simulink model "EsamblajeCohete2_0"  (R2023a)
settings: Solver=VariableStepAuto  StartTime=0.0  StopTime=15  RelTol=1e-3
model workspace: external: MATLAB File C:\Users\SEBASTIANDIAZPABON\OneDrive - Universidad Santo Tomás Bucaramanga\USTA\Semillero Cohete\Cohete Matlab 2.0\EsamblajeCohete2_0_DataFile.m (data not in the file)
undefined symbols (not defined in the file): smiData, X, Y, Z
libraries: sm_lib x355, nesl_utility x10, fuzblock x6, simulink x2
(part 1 of 7)
settings Model: SimulationMode=accelerator  Creator=SEBASTIANDIAZPABON  LastModifiedBy=kushkiclave1234
settings ModelReferenceCC: EnableRefExpFcnMdlSchedulingChecks=on

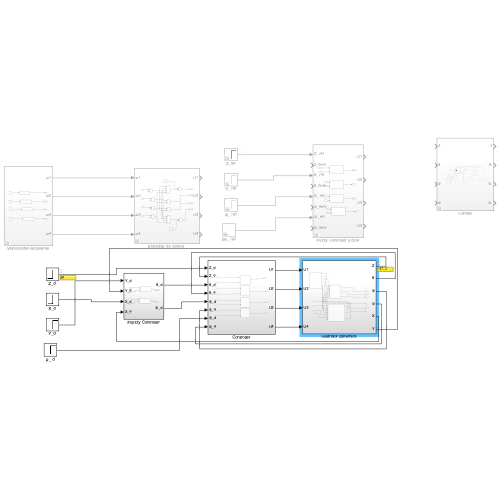
[thumbnail: Simulink's stored preview of the top-level diagram]
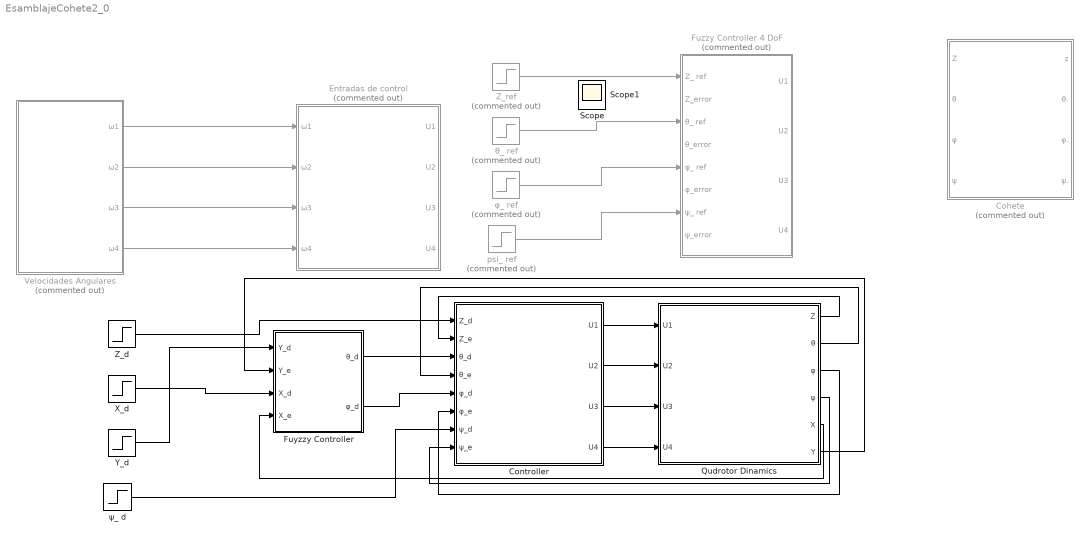
== system EsamblajeCohete2_0 ==
  Cohete : Subsystem  Commented=on
  Controller : Subsystem
  "Entradas de control " : Subsystem  Commented=on
  Fuyzzy Controller : Subsystem
  Fuzzy Controller 4 DoF : Subsystem  Commented=on
  Qudrotor Dinamics : Subsystem
  Velocidades Angulares : Subsystem  Commented=on
  X_d : Step  After=20  SampleTime=0
  Y_d : Step  After=20  SampleTime=0
  Z_d : Step  Time=0.01  After=30  SampleTime=0
  Z_ref : Step  Commented=on  Time=0  After=0  SampleTime=0
  psi_ ref : Step  Commented=on  Time=0  After=0.05  SampleTime=0
  θ_ ref : Step  Commented=on  Time=0  After=0.1  SampleTime=0
  φ_ ref : Step  Commented=on  Time=0  After=0.5  SampleTime=0
  ψ_ d : Step  After=20  SampleTime=0
  Scope : Scope
  Scope1 : Scope
  wires:
  Velocidades Angulares/1(ω1) -> "Entradas de control "/1(ω1)
  Velocidades Angulares/2(ω2) -> "Entradas de control "/2(ω2)
  Velocidades Angulares/3(ω3) -> "Entradas de control "/3(ω3)
  Velocidades Angulares/4(ω4) -> "Entradas de control "/4(ω4)
  Z_ref/1 -> Fuzzy Controller 4 DoF/1(Z_ ref)
  θ_ ref/1 -> Fuzzy Controller 4 DoF/3(θ_ ref)
  φ_ ref/1 -> Fuzzy Controller 4 DoF/5(φ_ ref)
  psi_ ref/1 -> Fuzzy Controller 4 DoF/7(ψ_ ref)
  Controller/1(U1) -> Qudrotor Dinamics/1(U1)
  Controller/2(U2) -> Qudrotor Dinamics/2(U2)
  Controller/3(U3) -> Qudrotor Dinamics/3(U3)
  Controller/4(U4) -> Qudrotor Dinamics/4(U4)
  Qudrotor Dinamics/1(Z) -> Controller/2(Z_e)
  Qudrotor Dinamics/2(θ) -> Controller/4(θ_e)
  Qudrotor Dinamics/3(φ) -> Controller/6(φ_e)
  Qudrotor Dinamics/4(ψ) -> Controller/8(ψ_e)
  Fuyzzy Controller/1(θ_d) -> Controller/3(θ_d)
  Qudrotor Dinamics/6(Y) -> Fuyzzy Controller/2(Y_e)
  Qudrotor Dinamics/5(X) -> Fuyzzy Controller/4(X_e)
  Fuyzzy Controller/2(φ_d) -> Controller/5(φ_d)
  Z_d/1 -> Controller/1(Z_d)
  X_d/1 -> Fuyzzy Controller/3(X_d)
  Y_d/1 -> Fuyzzy Controller/1(Y_d)
  ψ_ d/1 -> Controller/7(ψ_d)

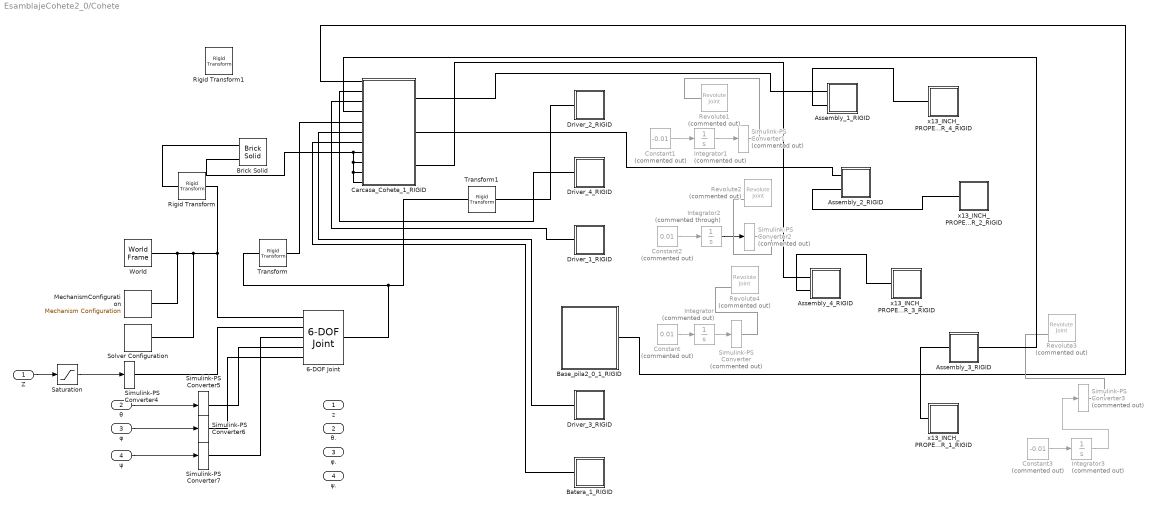
== system EsamblajeCohete2_0/Cohete ==
  Z : Inport
  θ : Inport  Port=2
  φ : Inport  Port=3
  ψ : Inport  Port=4
  6-DOF Joint : sm_lib/Joints/6-DOF Joint  JointMode=Normal  SenseConstraintForce=off  SenseConstraintForceX=off  SenseConstraintForceY=off  SenseConstraintForceZ=off  SenseConstraintTorque=off  SenseConstraintTorqueX=off  SenseConstraintTorqueY=off  SenseConstraintTorqueZ=off  SenseTotalForce=off  SenseTotalForceX=off  SenseTotalForceY=off  SenseTotalForceZ=off  SenseTotalTorque=off  SenseTotalTorqueX=off  SenseTotalTorqueY=off  SenseTotalTorqueZ=off  CompositeWrenchDir=FollowerOnBase  CompositeWrenchFrame=BaseFrame  PxEquilibriumPosition=0  PxEquilibriumPositionUnits=m  PxSpringStiffness=0  PxSpringStiffnessUnits=N/m  PxDampingCoefficient=0  PxDampingCoefficientUnits=N/(m/s)  PxTorqueActuationMode=NoTorque  PxMotionActuationMode=ComputedMotion  PxSensePosition=off  PxSenseVelocity=off  PxSenseAcceleration=off  PxSenseTorqueForce=off  PxSenseLowerLimitTorqueForce=off  PxSenseUpperLimitTorqueForce=off  PxLowerLimitSpecify=off  PxLowerLimitBound=-1  PxLowerLimitBoundUnits=m  PxLowerLimitStiffness=1e6  PxLowerLimitStiffnessUnits=N/m  PxLowerLimitDamping=1e3  PxLowerLimitDampingUnits=N/(m/s)  PxLowerLimitTransitionRegionWidth=1e-4  PxLowerLimitTransitionRegionWidthUnits=m  PxUpperLimitSpecify=off  PxUpperLimitBound=1  PxUpperLimitBoundUnits=m  PxUpperLimitStiffness=1e6  PxUpperLimitStiffnessUnits=N/m  PxUpperLimitDamping=1e3  PxUpperLimitDampingUnits=N/(m/s)  PxUpperLimitTransitionRegionWidth=1e-4  PxUpperLimitTransitionRegionWidthUnits=m  PxPositionTargetSpecify=off  PxPositionTargetPriority=High  PxPositionTargetValue=0  PxPositionTargetValueUnits=m  PxVelocityTargetSpecify=off  PxVelocityTargetPriority=High  PxVelocityTargetValue=0  PxVelocityTargetValueUnits=m/s  PyEquilibriumPosition=0  PyEquilibriumPositionUnits=m  PySpringStiffness=0  PySpringStiffnessUnits=N/m  PyDampingCoefficient=0  PyDampingCoefficientUnits=N/(m/s)  PyTorqueActuationMode=ComputedTorque  PyMotionActuationMode=InputMotion  PySensePosition=off  PySenseVelocity=off  PySenseAcceleration=off  PySenseTorqueForce=off  PySenseLowerLimitTorqueForce=off  PySenseUpperLimitTorqueForce=off  PyLowerLimitSpecify=on  PyLowerLimitBound=0  PyLowerLimitBoundUnits=m  PyLowerLimitStiffness=1e6  PyLowerLimitStiffnessUnits=N/m  PyLowerLimitDamping=1e3  PyLowerLimitDampingUnits=N/(m/s)  PyLowerLimitTransitionRegionWidth=1e-4  PyLowerLimitTransitionRegionWidthUnits=m  PyUpperLimitSpecify=off  PyUpperLimitBound=1  PyUpperLimitBoundUnits=m  PyUpperLimitStiffness=1e6  PyUpperLimitStiffnessUnits=N/m  PyUpperLimitDamping=1e3  PyUpperLimitDampingUnits=N/(m/s)  PyUpperLimitTransitionRegionWidth=1e-4  PyUpperLimitTransitionRegionWidthUnits=m  PyPositionTargetSpecify=off  PyPositionTargetPriority=High  PyPositionTargetValue=0  PyPositionTargetValueUnits=m  PyVelocityTargetSpecify=off  PyVelocityTargetPriority=High  PyVelocityTargetValue=0  PyVelocityTargetValueUnits=m/s  PzEquilibriumPosition=0  PzEquilibriumPositionUnits=m  PzSpringStiffness=0  PzSpringStiffnessUnits=N/m  PzDampingCoefficient=0  PzDampingCoefficientUnits=N/(m/s)  PzTorqueActuationMode=NoTorque  PzMotionActuationMode=ComputedMotion  PzSensePosition=off  PzSenseVelocity=off  PzSenseAcceleration=off  PzSenseTorqueForce=off  PzSenseLowerLimitTorqueForce=off  PzSenseUpperLimitTorqueForce=off  PzLowerLimitSpecify=off  PzLowerLimitBound=-1  PzLowerLimitBoundUnits=m  PzLowerLimitStiffness=1e6  PzLowerLimitStiffnessUnits=N/m  PzLowerLimitDamping=1e3  PzLowerLimitDampingUnits=N/(m/s)  PzLowerLimitTransitionRegionWidth=1e-4  PzLowerLimitTransitionRegionWidthUnits=m  PzUpperLimitSpecify=off  PzUpperLimitBound=1  PzUpperLimitBoundUnits=m  PzUpperLimitStiffness=1e6  PzUpperLimitStiffnessUnits=N/m  PzUpperLimitDamping=1e3  PzUpperLimitDampingUnits=N/(m/s)  PzUpperLimitTransitionRegionWidth=1e-4  PzUpperLimitTransitionRegionWidthUnits=m  PzPositionTargetSpecify=off  PzPositionTargetPriority=High  PzPositionTargetValue=0  PzPositionTargetValueUnits=m  PzVelocityTargetSpecify=off  PzVelocityTargetPriority=High  PzVelocityTargetValue=0  PzVelocityTargetValueUnits=m/s  SphEqPosRotationMethod=None  SphEqPosRotationAngleUnits=deg  SphEqPosRotationStandardAxis=+Z  SphEqPosRotationAngle=0.0  SphEqPosRotationArbitraryAxis=[0 0 1]  SphEqPosFollAlignAxisA=+X  SphEqPosBaseAlignAxisA=+Y  SphEqPosFollAlignAxisB=+Y  SphEqPosBaseAlignAxisB=+Z  SphEqPosRotationSequenceAxes=FollowerAxes  SphEqPosRotationSequence=XYX  SphEqPosRotationSequenceAngles=[0 0 0]  SphEqPosRotationSequenceAnglesUnits=deg  SphEqPosRotationMatrix=[1 0 0; 0 1 0; 0 0 1]  SphEqPosQuaternion=[1 0 0 0]  SphSpringStiffness=0  SphSpringStiffnessUnits=N*m/deg  SphDampingCoefficient=0  SphDampingCoefficientUnits=N*m/(deg/s)  SphActuateTorqueX=on  SphActuateTorqueY=on  SphActuateTorqueZ=on  SphActuateTorque=off  SphTorqueActuationMode=InputTorque  SphMotionActuationMode=ComputedMotion  SphActuationFrame=BaseFrame  SphSensePosition=off  SphSenseVelocityX=off  SphSenseVelocityY=off  SphSenseVelocityZ=off  SphSenseVelocity=off  SphSenseAccelerationX=off  SphSenseAccelerationY=off  SphSenseAccelerationZ=off  SphSenseAcceleration=off  SphSenseTorqueX=off  SphSenseTorqueY=off  SphSenseTorqueZ=off  SphSenseTorqueForce=off  SphSenseLowerLimitTorqueMag=off  SphSenseUpperLimitTorqueMag=off  SphSensingFrame=BaseFrame  SphLowerLimitSpecify=off  SphLowerLimitBound=15  SphLowerLimitBoundUnits=deg  SphLowerLimitStiffness=1e4  SphLowerLimitStiffnessUnits=N*m/deg  SphLowerLimitDamping=10  SphLowerLimitDampingUnits=N*m/(deg/s)  SphLowerLimitTransitionRegionWidth=0.1  SphLowerLimitTransitionRegionWidthUnits=deg  SphUpperLimitSpecify=off  SphUpperLimitBound=45  SphUpperLimitBoundUnits=deg  SphUpperLimitStiffness=1e4  SphUpperLimitStiffnessUnits=N*m/deg  SphUpperLimitDamping=10  SphUpperLimitDampingUnits=N*m/(deg/s)  SphUpperLimitTransitionRegionWidth=0.1  SphUpperLimitTransitionRegionWidthUnits=deg  SphPositionTargetRotationMethod=None  SphPositionTargetRotationAngleUnits=deg  SphPositionTargetRotationStandardAxis=+Z  SphPositionTargetRotationAngle=0.0  SphPositionTargetRotationArbitraryAxis=[0 0 1]  SphPositionTargetFollAlignAxisA=+X  SphPositionTargetBaseAlignAxisA=+Y  SphPositionTargetFollAlignAxisB=+Y  SphPositionTargetBaseAlignAxisB=+Z  SphPositionTargetRotationSequenceAxes=FollowerAxes  SphPositionTargetRotationSequence=XYX  SphPositionTargetRotationSequenceAngles=[0 0 0]  SphPositionTargetRotationSequenceAnglesUnits=deg  SphPositionTargetRotationMatrix=[1 0 0; 0 1 0; 0 0 1]  SphPositionTargetQuaternion=[1 0 0 0]  SphPositionTargetSpecify=off  SphPositionTargetPriority=High  SphVelocityTargetValue=[0 0 0]  SphVelocityTargetValueUnits=deg/s  SphVelocityTargetSpecify=off  SphVelocityTargetPriority=High  SphVelocityTargetInFollowerFrame=on
  Assembly_1_RIGID : Subsystem
  Assembly_2_RIGID : Subsystem
  Assembly_3_RIGID : Subsystem
  Assembly_4_RIGID : Subsystem
  Base_pila2_0_1_RIGID : Subsystem
  Batera_1_RIGID : Subsystem
  Brick Solid : sm_lib/Body Elements/Brick Solid  GraphicAmbientColor=[0.15 0.15 0.15 1.0]  BasedOnType=Density  BrickDimensions=[2 2 0.1 ]  BrickDimensionsUnits=m  CenterOfMass=[0 0 0]  CenterOfMassUnits=m  GraphicDiffuseColor=[0.4 0.6 0.0]  Density=1000  DensityUnits=kg/m^3  DoExposeReferenceFrame=on  GraphicEmissiveColor=[0.0 0.0 0.0 1.0]  ExportEntireGeometry=on  SerializedFrames=<Frames><Frame><Id>Frame1</Id><Value><Name>F1</Name><Origin><Source>ReferenceFrame</Source><FeatureName></FeatureName></Origin><PrimaryAxis><DefinedDirection>+Y</DefinedDirection><Source>ReferenceFrame</Source><SourceDirection>-Z</SourceDirection><FeatureName></FeatureName></PrimaryAxis><SecondaryAxis><DefinedDirection>+X</DefinedDirection><Source>ReferenceFrame</Source><SourceDirection>+X</SourceDirection><FeatureName></FeatureName></SecondaryAxis></Value></Frame></Frames>  MarkerShape=Sphere  MarkerSize=10  GraphicType=FromGeometry  InertiaType=CalculateFromGeometry  Mass=1  MassUnits=kg  MomentsOfInertia=[1 1 1]  MomentsOfInertiaUnits=kg*m^2  GraphicOpacity=1.0  ProductsOfInertia=[0 0 0]  ProductsOfInertiaUnits=kg*m^2  GraphicShininess=75  GraphicSpecularColor=[0.5 0.5 0.5 1.0]  GraphicVisPropType=SimpleVisualProperties
  Carcasa_Cohete_1_RIGID : Subsystem
  Constant : Constant  Commented=on  Value=0.01
  Constant1 : Constant  Commented=on  Value=-0.01
  Constant2 : Constant  Commented=on  Value=0.01
  Constant3 : Constant  Commented=on  Value=-0.01
  Driver_1_RIGID : Subsystem
  Driver_2_RIGID : Subsystem
  Driver_3_RIGID : Subsystem
  Driver_4_RIGID : Subsystem
  Integrator : Integrator  Commented=on
  Integrator1 : Integrator  Commented=on
  Integrator2 : Integrator  Commented=through
  Integrator3 : Integrator  Commented=on
  MechanismConfiguration : sm_lib/Utilities/Mechanism Configuration  UniformGravity=Constant  GravityVector=[0 0 0]  GravityVectorUnits=m/s^2  LinearizationDelta=0.001  JointModeTransitionNonlinearIterations=2
  Revolute1 : sm_lib/Joints/Revolute Joint  Commented=on  JointMode=Normal  SenseConstraintForce=off  SenseConstraintForceX=off  SenseConstraintForceY=off  SenseConstraintForceZ=off  SenseConstraintTorque=off  SenseConstraintTorqueX=off  SenseConstraintTorqueY=off  SenseConstraintTorqueZ=off  SenseTotalForce=off  SenseTotalForceX=off  SenseTotalForceY=off  SenseTotalForceZ=off  SenseTotalTorque=off  SenseTotalTorqueX=off  SenseTotalTorqueY=off  SenseTotalTorqueZ=off  CompositeWrenchDir=FollowerOnBase  CompositeWrenchFrame=BaseFrame  EquilibriumPosition=0  EquilibriumPositionUnits=deg  SpringStiffness=0  SpringStiffnessUnits=N*m/deg  DampingCoefficient=0  DampingCoefficientUnits=N*m/(deg/s)  TorqueActuationMode=InputTorque  MotionActuationMode=InputMotion  SensePosition=off  SenseVelocity=off  SenseAcceleration=off  SenseTorqueForce=off  SenseLowerLimitTorqueForce=off  SenseUpperLimitTorqueForce=off  LowerLimitSpecify=off  LowerLimitBound=-90  LowerLimitBoundUnits=deg  LowerLimitStiffness=1e4  LowerLimitStiffnessUnits=N*m/deg  LowerLimitDamping=10  LowerLimitDampingUnits=N*m/(deg/s)  LowerLimitTransitionRegionWidth=0.1  LowerLimitTransitionRegionWidthUnits=deg  UpperLimitSpecify=off  UpperLimitBound=90  UpperLimitBoundUnits=deg  UpperLimitStiffness=1e4  UpperLimitStiffnessUnits=N*m/deg  UpperLimitDamping=10  UpperLimitDampingUnits=N*m/(deg/s)  UpperLimitTransitionRegionWidth=0.1  UpperLimitTransitionRegionWidthUnits=deg  PositionTargetSpecify=on  PositionTargetPriority=Low  PositionTargetValue=smiData.RevoluteJoint(2).Rz.Pos  PositionTargetValueUnits=deg  VelocityTargetSpecify=off  VelocityTargetPriority=High  VelocityTargetValue=0  VelocityTargetValueUnits=deg/s
  Revolute2 : sm_lib/Joints/Revolute Joint  Commented=on  JointMode=Normal  SenseConstraintForce=off  SenseConstraintForceX=off  SenseConstraintForceY=off  SenseConstraintForceZ=off  SenseConstraintTorque=off  SenseConstraintTorqueX=off  SenseConstraintTorqueY=off  SenseConstraintTorqueZ=off  SenseTotalForce=off  SenseTotalForceX=off  SenseTotalForceY=off  SenseTotalForceZ=off  SenseTotalTorque=off  SenseTotalTorqueX=off  SenseTotalTorqueY=off  SenseTotalTorqueZ=off  CompositeWrenchDir=FollowerOnBase  CompositeWrenchFrame=BaseFrame  EquilibriumPosition=0  EquilibriumPositionUnits=deg  SpringStiffness=0  SpringStiffnessUnits=N*m/deg  DampingCoefficient=0  DampingCoefficientUnits=N*m/(deg/s)  TorqueActuationMode=InputTorque  MotionActuationMode=ComputedMotion  SensePosition=off  SenseVelocity=off  SenseAcceleration=off  SenseTorqueForce=off  SenseLowerLimitTorqueForce=off  SenseUpperLimitTorqueForce=off  LowerLimitSpecify=off  LowerLimitBound=-90  LowerLimitBoundUnits=deg  LowerLimitStiffness=1e4  LowerLimitStiffnessUnits=N*m/deg  LowerLimitDamping=10  LowerLimitDampingUnits=N*m/(deg/s)  LowerLimitTransitionRegionWidth=0.1  LowerLimitTransitionRegionWidthUnits=deg  UpperLimitSpecify=off  UpperLimitBound=90  UpperLimitBoundUnits=deg  UpperLimitStiffness=1e4  UpperLimitStiffnessUnits=N*m/deg  UpperLimitDamping=10  UpperLimitDampingUnits=N*m/(deg/s)  UpperLimitTransitionRegionWidth=0.1  UpperLimitTransitionRegionWidthUnits=deg  PositionTargetSpecify=on  PositionTargetPriority=Low  PositionTargetValue=smiData.RevoluteJoint(3).Rz.Pos  PositionTargetValueUnits=deg  VelocityTargetSpecify=off  VelocityTargetPriority=High  VelocityTargetValue=0  VelocityTargetValueUnits=deg/s
  Revolute3 : sm_lib/Joints/Revolute Joint  Commented=on  JointMode=Normal  SenseConstraintForce=off  SenseConstraintForceX=off  SenseConstraintForceY=off  SenseConstraintForceZ=off  SenseConstraintTorque=off  SenseConstraintTorqueX=off  SenseConstraintTorqueY=off  SenseConstraintTorqueZ=off  SenseTotalForce=off  SenseTotalForceX=off  SenseTotalForceY=off  SenseTotalForceZ=off  SenseTotalTorque=off  SenseTotalTorqueX=off  SenseTotalTorqueY=off  SenseTotalTorqueZ=off  CompositeWrenchDir=FollowerOnBase  CompositeWrenchFrame=BaseFrame  EquilibriumPosition=0  EquilibriumPositionUnits=deg  SpringStiffness=0  SpringStiffnessUnits=N*m/deg  DampingCoefficient=0  DampingCoefficientUnits=N*m/(deg/s)  TorqueActuationMode=InputTorque  MotionActuationMode=ComputedMotion  SensePosition=off  SenseVelocity=off  SenseAcceleration=off  SenseTorqueForce=off  SenseLowerLimitTorqueForce=off  SenseUpperLimitTorqueForce=off  LowerLimitSpecify=off  LowerLimitBound=-90  LowerLimitBoundUnits=deg  LowerLimitStiffness=1e4  LowerLimitStiffnessUnits=N*m/deg  LowerLimitDamping=10  LowerLimitDampingUnits=N*m/(deg/s)  LowerLimitTransitionRegionWidth=0.1  LowerLimitTransitionRegionWidthUnits=deg  UpperLimitSpecify=off  UpperLimitBound=90  UpperLimitBoundUnits=deg  UpperLimitStiffness=1e4  UpperLimitStiffnessUnits=N*m/deg  UpperLimitDamping=10  UpperLimitDampingUnits=N*m/(deg/s)  UpperLimitTransitionRegionWidth=0.1  UpperLimitTransitionRegionWidthUnits=deg  PositionTargetSpecify=on  PositionTargetPriority=Low  PositionTargetValue=smiData.RevoluteJoint(4).Rz.Pos  PositionTargetValueUnits=deg  VelocityTargetSpecify=off  VelocityTargetPriority=High  VelocityTargetValue=0  VelocityTargetValueUnits=deg/s
  Revolute4 : sm_lib/Joints/Revolute Joint  Commented=on  JointMode=Normal  SenseConstraintForce=off  SenseConstraintForceX=off  SenseConstraintForceY=off  SenseConstraintForceZ=off  SenseConstraintTorque=off  SenseConstraintTorqueX=off  SenseConstraintTorqueY=off  SenseConstraintTorqueZ=off  SenseTotalForce=off  SenseTotalForceX=off  SenseTotalForceY=off  SenseTotalForceZ=off  SenseTotalTorque=off  SenseTotalTorqueX=off  SenseTotalTorqueY=off  SenseTotalTorqueZ=off  CompositeWrenchDir=FollowerOnBase  CompositeWrenchFrame=BaseFrame  EquilibriumPosition=0  EquilibriumPositionUnits=deg  SpringStiffness=0  SpringStiffnessUnits=N*m/deg  DampingCoefficient=0  DampingCoefficientUnits=N*m/(deg/s)  TorqueActuationMode=InputTorque  MotionActuationMode=ComputedMotion  SensePosition=off  SenseVelocity=off  SenseAcceleration=off  SenseTorqueForce=off  SenseLowerLimitTorqueForce=off  SenseUpperLimitTorqueForce=off  LowerLimitSpecify=off  LowerLimitBound=-90  LowerLimitBoundUnits=deg  LowerLimitStiffness=1e4  LowerLimitStiffnessUnits=N*m/deg  LowerLimitDamping=10  LowerLimitDampingUnits=N*m/(deg/s)  LowerLimitTransitionRegionWidth=0.1  LowerLimitTransitionRegionWidthUnits=deg  UpperLimitSpecify=off  UpperLimitBound=90  UpperLimitBoundUnits=deg  UpperLimitStiffness=1e4  UpperLimitStiffnessUnits=N*m/deg  UpperLimitDamping=10  UpperLimitDampingUnits=N*m/(deg/s)  UpperLimitTransitionRegionWidth=0.1  UpperLimitTransitionRegionWidthUnits=deg  PositionTargetSpecify=on  PositionTargetPriority=Low  PositionTargetValue=smiData.RevoluteJoint(5).Rz.Pos  PositionTargetValueUnits=deg  VelocityTargetSpecify=off  VelocityTargetPriority=High  VelocityTargetValue=0  VelocityTargetValueUnits=deg/s
  Rigid Transform : sm_lib/Frames and Transforms/Rigid Transform  TranslationMethod=Cartesian  TranslationStandardOffset=0  TranslationStandardOffsetUnits=m  TranslationStandardAxis=+Z  TranslationCartesianOffset=[0 0.28 0]  TranslationCartesianOffsetUnits=m  TranslationROffset=0  TranslationROffsetUnits=m  TranslationZOffset=0  TranslationZOffsetUnits=m  TranslationThetaOffset=0  TranslationThetaOffsetUnits=deg  RotationMethod=None  RotationAngleUnits=deg  RotationStandardAxis=+Z  RotationAngle=0.0  RotationArbitraryAxis=[0 0 1]  FollAlignAxisA=+X  BaseAlignAxisA=+Y  FollAlignAxisB=+Y  BaseAlignAxisB=+Z  RotationSequenceAxes=FollowerAxes  RotationSequence=XYX  RotationSequenceAngles=[0 0 0]  RotationSequenceAnglesUnits=deg  RotationMatrix=[1 0 0; 0 1 0; 0 0 1]  Quaternion=[1 0 0 0]
  Rigid Transform1 : sm_lib/Frames and Transforms/Rigid Transform  TranslationMethod=None  TranslationStandardOffset=0  TranslationStandardOffsetUnits=m  TranslationStandardAxis=+Z  TranslationCartesianOffset=[0 0 0]  TranslationCartesianOffsetUnits=m  TranslationROffset=0  TranslationROffsetUnits=m  TranslationZOffset=0  TranslationZOffsetUnits=m  TranslationThetaOffset=0  TranslationThetaOffsetUnits=deg  RotationMethod=None  RotationAngleUnits=deg  RotationStandardAxis=+Z  RotationAngle=0.0  RotationArbitraryAxis=[0 0 1]  FollAlignAxisA=+X  BaseAlignAxisA=+Y  FollAlignAxisB=+Y  BaseAlignAxisB=+Z  RotationSequenceAxes=FollowerAxes  RotationSequence=XYX  RotationSequenceAngles=[0 0 0]  RotationSequenceAnglesUnits=deg  RotationMatrix=[1 0 0; 0 1 0; 0 0 1]  Quaternion=[1 0 0 0]
  Saturation : Saturate  UpperLimit=2  LowerLimit=-2
  Simulink-PS Converter{,1..3} (4 alike) : nesl_utility/Simulink-PS Converter  Commented=on  PhysicalDomain=network_engine_domain  SubClassName=ps_input  LeftPortType=input  RightPortType=output  PseudoPeriodic=off  Frequencies=[]  NoiseDistribution=none  NoiseParameters=[]  Unit=1  AffineConversion=off  FilteringAndDerivatives=filter  SimscapeFilterOrder=2  InputFilterTimeConstant=0.001  UdotUserProvided=0
  Simulink-PS Converter{4..7} (4 alike) : nesl_utility/Simulink-PS Converter  PhysicalDomain=network_engine_domain  SubClassName=ps_input  LeftPortType=input  RightPortType=output  PseudoPeriodic=off  Frequencies=[]  NoiseDistribution=none  NoiseParameters=[]  Unit=1  AffineConversion=off  FilteringAndDerivatives=filter  SimscapeFilterOrder=2  InputFilterTimeConstant=0.001  UdotUserProvided=0
  Solver Configuration : nesl_utility/Solver Configuration  PhysicalDomain=network_engine_domain  SubClassName=solver  LeftPortType=input  RightPortType=generic  Tones=[]  Harmonics=[]  SimulateNoise=off  Profile=off  UseLocalSampling=off  EnableSwitchedLinearOptims=on  FrequencyDomain=off  UseCCode=off  RelTol=0.001  AbsTol=0.001  MinStep=1e-09  ToWorkspace=off  RevertToSquareIcSolve=off  NumHomotopyIterations=100  PhasorMode=off  PhasorModeNumHarmonics=1  ConsistencySolver=NEWTON_FTOL  IndexReductionMethod=DerivativeReplacement  DoDC=off  ResidualTolerance=1e-09  ConsistencyTolSource=GLOBAL  ConsistencyAbsTol=0.001  ConsistencyRelTol=0.001  ConsistencyTolFactor=0.001  UseLocalSolver=off  LocalSolverChoice=NE_BACKWARD_EULER_ADVANCER  ResolveIndetEquations=on  FunctionEvalNumThread=1  LocalSolverSampleTime=0.001  DoFixedCost=off  MaxNonlinIter=3  MaxModeIter=2  ComputeImpulses=off  ImpulseIterations=2  LinearAlgebra=auto  LinearAlgebraNumThread=0  EquationFormulation=NE_TIME_EF  DelaysMemoryBudget=1024  AutomaticFiltering=on  FilteringTimeConstant=0.001  PartitionStorageMethod=AS_NEEDED  PartitionMemoryBudget=1024  PartitionMethod=ROBUST
  Transform : sm_lib/Frames and Transforms/Rigid Transform  TranslationMethod=Cartesian  TranslationStandardOffset=0  TranslationStandardOffsetUnits=mm  TranslationStandardAxis=+Z  TranslationCartesianOffset=smiData.RigidTransform(12).translation  TranslationCartesianOffsetUnits=mm  TranslationROffset=0  TranslationROffsetUnits=m  TranslationZOffset=0  TranslationZOffsetUnits=m  TranslationThetaOffset=0  TranslationThetaOffsetUnits=deg  RotationMethod=ArbitraryAxis  RotationAngleUnits=rad  RotationStandardAxis=+Z  RotationAngle=smiData.RigidTransform(12).angle  RotationArbitraryAxis=smiData.RigidTransform(12).axis  FollAlignAxisA=+X  BaseAlignAxisA=+Y  FollAlignAxisB=+Y  BaseAlignAxisB=+Z  RotationSequenceAxes=FollowerAxes  RotationSequence=XYX  RotationSequenceAngles=[0 0 0]  RotationSequenceAnglesUnits=deg  RotationMatrix=[1 0 0; 0 1 0; 0 0 1]  Quaternion=[1 0 0 0]
  Transform1 : sm_lib/Frames and Transforms/Rigid Transform  TranslationMethod=Cartesian  TranslationStandardOffset=0  TranslationStandardOffsetUnits=mm  TranslationStandardAxis=+Z  TranslationCartesianOffset=smiData.RigidTransform(123).translation  TranslationCartesianOffsetUnits=mm  TranslationROffset=0  TranslationROffsetUnits=m  TranslationZOffset=0  TranslationZOffsetUnits=m  TranslationThetaOffset=0  TranslationThetaOffsetUnits=deg  RotationMethod=ArbitraryAxis  RotationAngleUnits=rad  RotationStandardAxis=+Z  RotationAngle=smiData.RigidTransform(123).angle  RotationArbitraryAxis=smiData.RigidTransform(123).axis  FollAlignAxisA=+X  BaseAlignAxisA=+Y  FollAlignAxisB=+Y  BaseAlignAxisB=+Z  RotationSequenceAxes=FollowerAxes  RotationSequence=XYX  RotationSequenceAngles=[0 0 0]  RotationSequenceAnglesUnits=deg  RotationMatrix=[1 0 0; 0 1 0; 0 0 1]  Quaternion=[1 0 0 0]
  World : sm_lib/Frames and Transforms/World Frame
  x13_INCH_PROPELLER_1_RIGID : Subsystem
  x13_INCH_PROPELLER_2_RIGID : Subsystem
  x13_INCH_PROPELLER_3_RIGID : Subsystem
  x13_INCH_PROPELLER_4_RIGID : Subsystem
  z : Outport
  θ. : Outport  Port=2
  φ. : Outport  Port=3
  ψ. : Outport  Port=4
  wires:
  θ/1 -> Simulink-PS Converter5/1
  φ/1 -> Simulink-PS Converter6/1
  Z/1 -> Saturation/1
  Integrator3/1 -> Simulink-PS Converter3/1
  Integrator1/1 -> Simulink-PS Converter1/1
  Integrator2/1 -> Simulink-PS Converter2/1
  Constant3/1 -> Integrator3/1
  Constant/1 -> Integrator/1
  Constant1/1 -> Integrator1/1
  Constant2/1 -> Integrator2/1
  Integrator/1 -> Simulink-PS Converter/1
  ψ/1 -> Simulink-PS Converter7/1
  Saturation/1 -> Simulink-PS Converter4/1
  connections:
  Driver_2_RIGID/LConn1 -- Transform1/RConn1
  Assembly_3_RIGID/LConn1 -- x13_INCH_PROPELLER_1_RIGID/LConn1
  Revolute1/LConn2 -- Simulink-PS Converter1/RConn1
  Transform/RConn1 -- Carcasa_Cohete_1_RIGID/LConn5
  Base_pila2_0_1_RIGID/RConn1 -- Carcasa_Cohete_1_RIGID/LConn1
  Assembly_4_RIGID/LConn2 -- x13_INCH_PROPELLER_3_RIGID/LConn1
  Simulink-PS Converter2/RConn1 -- Revolute2/LConn2
  Revolute3/LConn2 -- Simulink-PS Converter3/RConn1
  Transform1/LConn1 -- Transform/LConn1 -- 6-DOF Joint/RConn1
  Simulink-PS Converter/RConn1 -- Revolute4/LConn2
  Batera_1_RIGID/LConn1 -- Carcasa_Cohete_1_RIGID/LConn7
  Assembly_1_RIGID/LConn2 -- x13_INCH_PROPELLER_4_RIGID/LConn1
  Driver_4_RIGID/LConn1 -- Carcasa_Cohete_1_RIGID/LConn2
  Driver_3_RIGID/LConn1 -- Carcasa_Cohete_1_RIGID/LConn6
  Driver_1_RIGID/LConn1 -- Carcasa_Cohete_1_RIGID/LConn3
  Assembly_2_RIGID/LConn2 -- x13_INCH_PROPELLER_2_RIGID/LConn1
  Brick Solid/LConn2 -- Carcasa_Cohete_1_RIGID/LConn11 -- Carcasa_Cohete_1_RIGID/LConn10 -- Carcasa_Cohete_1_RIGID/LConn9 -- Carcasa_Cohete_1_RIGID/LConn8
  Simulink-PS Converter4/RConn1 -- 6-DOF Joint/LConn2
  Carcasa_Cohete_1_RIGID/RConn2 -- Assembly_2_RIGID/LConn1
  Carcasa_Cohete_1_RIGID/RConn1 -- Assembly_1_RIGID/LConn1
  Carcasa_Cohete_1_RIGID/RConn3 -- Assembly_4_RIGID/LConn1
  Carcasa_Cohete_1_RIGID/LConn4 -- Assembly_3_RIGID/RConn1
  MechanismConfiguration/RConn1 -- World/RConn1 -- Rigid Transform/RConn1 -- 6-DOF Joint/LConn1 -- Solver Configuration/RConn1
  Rigid Transform/LConn1 -- Brick Solid/LConn1
  Simulink-PS Converter7/RConn1 -- 6-DOF Joint/LConn3
  Simulink-PS Converter5/RConn1 -- 6-DOF Joint/LConn4
  Simulink-PS Converter6/RConn1 -- 6-DOF Joint/LConn5

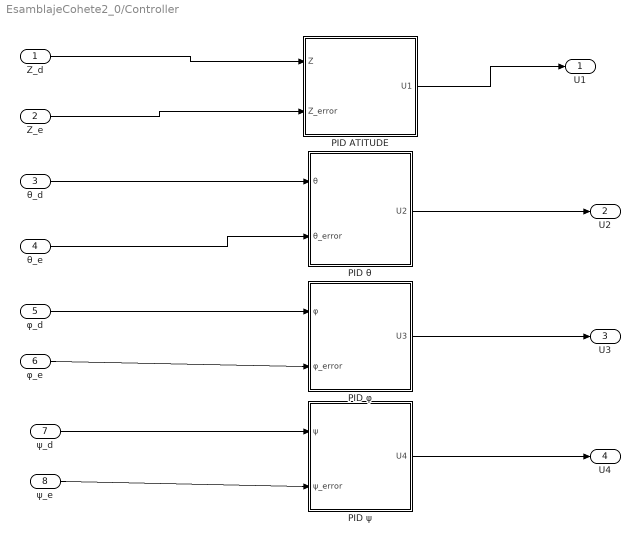
== system EsamblajeCohete2_0/Controller ==
  Z_d : Inport
  Z_e : Inport  Port=2
  θ_d : Inport  Port=3
  θ_e : Inport  Port=4
  φ_d : Inport  Port=5
  φ_e : Inport  Port=6
  ψ_d : Inport  Port=7
  ψ_e : Inport  Port=8
  PID ATITUDE : Subsystem
  "PID θ   " : Subsystem
  PID φ : Subsystem
  PID ψ : Subsystem
  U1 : Outport
  U2 : Outport  Port=2
  U3 : Outport  Port=3
  U4 : Outport  Port=4
  wires:
  PID ATITUDE/1(U1) -> U1/1
  "PID θ   "/1(U2) -> U2/1
  Z_d/1 -> PID ATITUDE/1(Z)
  Z_e/1 -> PID ATITUDE/2(Z_error)
  θ_d/1 -> "PID θ   "/1(θ)
  θ_e/1 -> "PID θ   "/2(θ_error)
  φ_d/1 -> PID φ/1(φ)
  φ_e/1 -> PID φ/2(φ_error)
  PID φ/1(U3) -> U3/1
  PID ψ/1(U4) -> U4/1
  ψ_d/1 -> PID ψ/1(ψ)
  ψ_e/1 -> PID ψ/2(ψ_error)

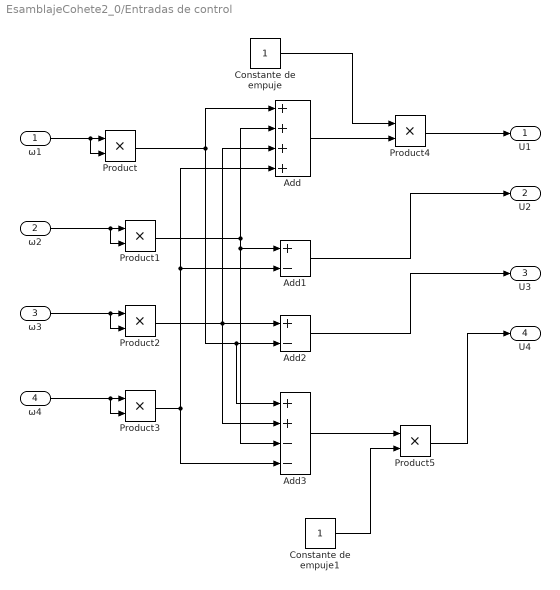
== system EsamblajeCohete2_0/Entradas de control  ==
  ω1 : Inport
  ω2 : Inport  Port=2
  ω3 : Inport  Port=3
  ω4 : Inport  Port=4
  Add : Sum  Inputs=++++
  Add1 : Sum  Inputs=+-
  Add2 : Sum  Inputs=+-
  Add3 : Sum  Inputs=++--
  Constante de empuje : Constant
  Constante de empuje1 : Constant
  Product{,1..5} (6 alike) : Product
  U1 : Outport
  U2 : Outport  Port=2
  U3 : Outport  Port=3
  U4 : Outport  Port=4
  wires:
  ω1/1 -> Product/2, Product/1
  ω2/1 -> Product1/2, Product1/1
  ω3/1 -> Product2/2, Product2/1
  ω4/1 -> Product3/2, Product3/1
  Product/1 -> Add3/1, Add2/2, Add/1
  Product1/1 -> Add1/1, Add3/3, Add/2
  Product2/1 -> Add2/1, Add/3, Add3/2
  Product3/1 -> Add3/4, Add1/2, Add/4
  Add/1 -> Product4/2
  Constante de empuje/1 -> Product4/1
  Product4/1 -> U1/1
  Add1/1 -> U2/1
  Add2/1 -> U3/1
  Add3/1 -> Product5/1
  Constante de empuje1/1 -> Product5/2
  Product5/1 -> U4/1

== system EsamblajeCohete2_0/Fuyzzy Controller ==
  Y_d : Inport
  Y_e : Inport  Port=2
  X_d : Inport  Port=3
  X_e : Inport  Port=4
  Fuzzy Lateral Controller : Subsystem
  Fuzzy Longitudinal Controller : Subsystem
  θ_d : Outport
  φ_d : Outport  Port=2
  wires:
  Y_d/1 -> Fuzzy Longitudinal Controller/1(Y_d)
  Fuzzy Longitudinal Controller/1(θ_d) -> θ_d/1
  Y_e/1 -> Fuzzy Longitudinal Controller/2(Y_e)
  X_d/1 -> Fuzzy Lateral Controller/1(X_d)
  Fuzzy Lateral Controller/1(θ_d) -> φ_d/1
  X_e/1 -> Fuzzy Lateral Controller/2(X_e)

== system EsamblajeCohete2_0/Fuzzy Controller 4 DoF ==
  Z_ ref : Inport
  Z_error : Inport  Port=2
  θ_ ref : Inport  Port=3
  θ_error : Inport  Port=4
  φ_ ref : Inport  Port=5
  φ_error : Inport  Port=6
  ψ_ ref : Inport  Port=7
  ψ_error : Inport  Port=8
  Fuzzy Controller Z : Subsystem
  Fuzzy Controller θ : Subsystem
  Fuzzy Controller φ : Subsystem
  Fuzzy Controller ψ : Subsystem
  U1 : Outport
  U2 : Outport  Port=2
  U3 : Outport  Port=3
  U4 : Outport  Port=4
  wires:
  ψ_ ref/1 -> Fuzzy Controller ψ/1(ψ_ ref)
  θ_error/1 -> Fuzzy Controller θ/2(θ_error)
  ψ_error/1 -> Fuzzy Controller ψ/2(ψ_error)
  φ_error/1 -> Fuzzy Controller φ/2(φ_error)
  θ_ ref/1 -> Fuzzy Controller θ/1(θ_ ref)
  Fuzzy Controller ψ/1(U4) -> U4/1
  φ_ ref/1 -> Fuzzy Controller φ/1(φ_ ref)
  Z_ ref/1 -> Fuzzy Controller Z/1(Z_ ref)
  Z_error/1 -> Fuzzy Controller Z/2(Z_error)
  Fuzzy Controller Z/1(U1) -> U1/1
  Fuzzy Controller θ/1(U3) -> U3/1
  Fuzzy Controller φ/1(U2) -> U2/1

== system EsamblajeCohete2_0/Qudrotor Dinamics ==
  U1 : Inport
  U2 : Inport  Port=2
  U3 : Inport  Port=3
  U4 : Inport  Port=4
  Constantes : Subsystem
  Rotacional : Subsystem
  Traslacional : Subsystem
  Z : Outport
  θ : Outport  Port=2
  φ : Outport  Port=3
  ψ : Outport  Port=4
  X : Outport  Port=5
  Y : Outport  Port=6
  wires:
  Constantes/2(g) -> Traslacional/1(g)
  Constantes/3(m) -> Traslacional/3(m)
  U1/1 -> Traslacional/2(U1)
  Traslacional/1(Z) -> Z/1
  Constantes/4(Ixx) -> Rotacional/1(Ixx)
  Constantes/5(Iyy) -> Rotacional/2(Iyy)
  Constantes/6(Izz) -> Rotacional/3(Izz)
  Constantes/1(l) -> Rotacional/7(L)
  U2/1 -> Rotacional/4(U2)
  U3/1 -> Rotacional/5(U3)
  U4/1 -> Rotacional/6(U4)
  Rotacional/1(θ) -> Traslacional/4(θ), θ/1
  Rotacional/2(φ) -> Traslacional/6(φ), φ/1
  Rotacional/3(ψ) -> Traslacional/5(ψ), ψ/1
  Traslacional/2(X) -> X/1
  Traslacional/3(Y) -> Y/1

== system EsamblajeCohete2_0/Velocidades Angulares ==
  Step{,1..3} (4 alike) : Step  Time=0.12  After=5  SampleTime=0
  Transfer Fcn{,1..3} (4 alike) : TransferFcn  Numerator=[0.15]  Denominator=[0.0000023 0.0001 0.002683]
  ω1 : Outport
  ω2 : Outport  Port=2
  ω3 : Outport  Port=3
  ω4 : Outport  Port=4
  wires:
  Transfer Fcn/1 -> ω1/1
  Transfer Fcn1/1 -> ω2/1
  Transfer Fcn2/1 -> ω3/1
  Transfer Fcn3/1 -> ω4/1
  Step/1 -> Transfer Fcn/1
  Step1/1 -> Transfer Fcn1/1
  Step2/1 -> Transfer Fcn2/1
  Step3/1 -> Transfer Fcn3/1
